simulink model "DSSS_spectrum_analysis"  (R2016a)
settings: Solver=VariableStepAuto  StartTime=0.0  StopTime=2  RelTol=1e-3
libraries: dspfdesign x2, commutil2 x2, commseqgen3 x1, commrandsrc3 x1
settings Model: Creator=malaika  LastModifiedBy=malaika

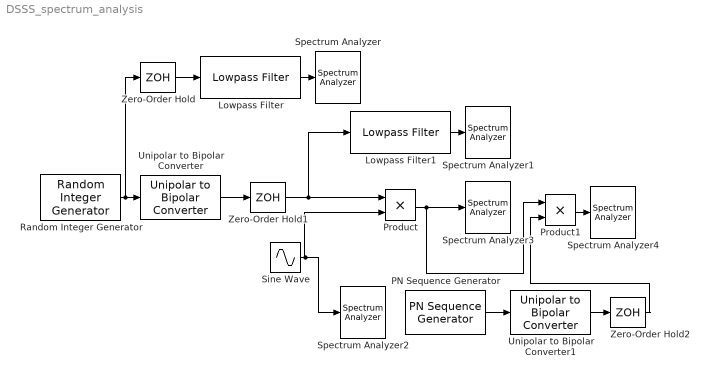
== system DSSS_spectrum_analysis ==
  Lowpass Filter : dspfdesign/Lowpass Filter  FilterType=FIR  DesignForMinimumOrder=on  FilterOrder=50  PassbandFrequency=400  StopbandFrequency=500  PassbandRipple=0.1  StopbandAttenuation=80  InheritSampleRate=on  SampleRate=44100  roundingMode=Floor  coeffsDataTypeStr=fixdt(1,16)  SimulateUsing=Interpreted execution
  Lowpass Filter1 : dspfdesign/Lowpass Filter  FilterType=FIR  DesignForMinimumOrder=on  FilterOrder=50  PassbandFrequency=400  StopbandFrequency=500  PassbandRipple=0.1  StopbandAttenuation=80  InheritSampleRate=on  SampleRate=44100  roundingMode=Floor  coeffsDataTypeStr=fixdt(1,16)  SimulateUsing=Interpreted execution
  PN Sequence Generator : commseqgen3/PN Sequence Generator  poly='z^10 + z^3 + 1'  ini_sta=[0 0 0 0 0 0 0 0 0 1]  outBitMaskSource=Dialog parameter  shift=0  outVarSiz=off  maxOutSizeMode=Dialog parameter  maxOutSize=[10 1]  Ts=0.0002  sampPerFrame=1  reset=off  bitPackedOutputs=off  outDataType=double  numPackedBits=8  bitPackDataSigned=off  bitPackedOutDType=double
  Product : Product
  Product1 : Product
  Random Integer Generator : commrandsrc3/Random Integer Generator  SetSize=2  SeedSource=Auto  Seed=0  SampleTime=0.002  SamplesPerFrame=1  OutputDataType=double  SimulateUsing=Interpreted execution
  Sine Wave : Sin  Frequency=2*pi*5000  SampleTime=0.00002
  Spectrum Analyzer{,1..4} (5 alike) : SpectrumAnalyzer
  Unipolar to Bipolar Converter : commutil2/Unipolar to Bipolar Converter  M=2  polarity=Positive  dataType=Inherit via internal rule
  Unipolar to Bipolar Converter1 : commutil2/Unipolar to Bipolar Converter  M=2  polarity=Positive  dataType=Inherit via internal rule
  Zero-Order Hold : ZeroOrderHold  SampleTime=0.00002
  Zero-Order Hold1 : ZeroOrderHold  SampleTime=0.00002
  Zero-Order Hold2 : ZeroOrderHold  SampleTime=0.00002
  wires:
  Random Integer Generator/1 -> Unipolar to Bipolar Converter/1, Zero-Order Hold/1
  Zero-Order Hold/1 -> Lowpass Filter/1
  Lowpass Filter/1 -> Spectrum Analyzer/1
  Unipolar to Bipolar Converter/1 -> Zero-Order Hold1/1
  Lowpass Filter1/1 -> Spectrum Analyzer1/1
  Sine Wave/1 -> Spectrum Analyzer2/1, Product/2
  Zero-Order Hold1/1 -> Lowpass Filter1/1, Product/1
  Product/1 -> Product1/1, Spectrum Analyzer3/1
  Zero-Order Hold2/1 -> Product1/2
  Product1/1 -> Spectrum Analyzer4/1
  PN Sequence Generator/1 -> Unipolar to Bipolar Converter1/1
  Unipolar to Bipolar Converter1/1 -> Zero-Order Hold2/1
